simulink model "progetto_sim"  (R2025b)
settings: Solver=VariableStepAuto  StartTime=0.0  StopTime=1000  RelTol=1e-3
values from neighbouring files (symbols this model uses):
  d0 = [110 130 100 160]    [backup_id_macchine.mat]    (also in id_macchine.mat)
  dmin = 4    [backup_id_macchine.mat]    (also in id_macchine.mat)
  mDist = [156.727602966 155.419177889 157.307233343 156.111472907]    [backup_id_macchine.mat]    (also in id_macchine.mat = [156.911734511 155.758692096 157.721037406 156.538222818])
  t_cth = 3    [backup_id_macchine.mat]    (also in id_macchine.mat)
  Ts = 2    [backup_id_macchine.mat]    (also in id_macchine.mat)
  umax = 600    [backup_id_macchine.mat]    (also in id_macchine.mat)
  umin = -600    [backup_id_macchine.mat]    (also in id_macchine.mat)
  v0 = [10 12 15 9 10]    [backup_id_macchine.mat]    (also in id_macchine.mat)
  vMedio = [9.99088198605 9.9851530035 9.98261849858 9.98180014012]    [backup_id_macchine.mat]    (also in id_macchine.mat = [10.0026522625 10.0031571294 10.0027874656 10.0025052689])
  x0 = [10 12 15 9 10]    [backup_id_macchine.mat]    (also in id_macchine.mat)
undefined symbols (not defined in the file or in its folder): d1, d2, d3, d4, dspblkCoreblockFVToolHelper, gcbh, s2v2, s3v2, s4v2, s5v2
libraries: simulink x3, slctrl_signal x1
settings Model: Creator=david  LastModifiedBy=david

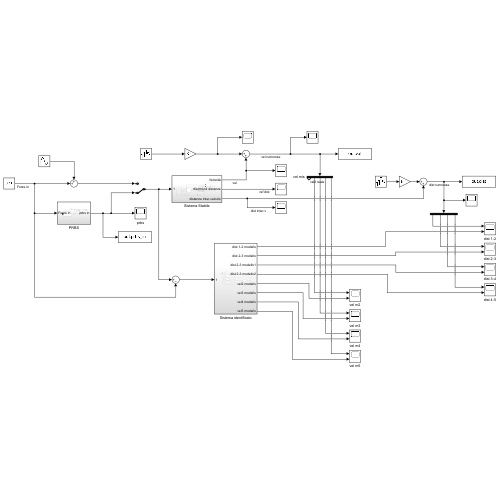
[thumbnail: Simulink's stored preview of the top-level diagram]
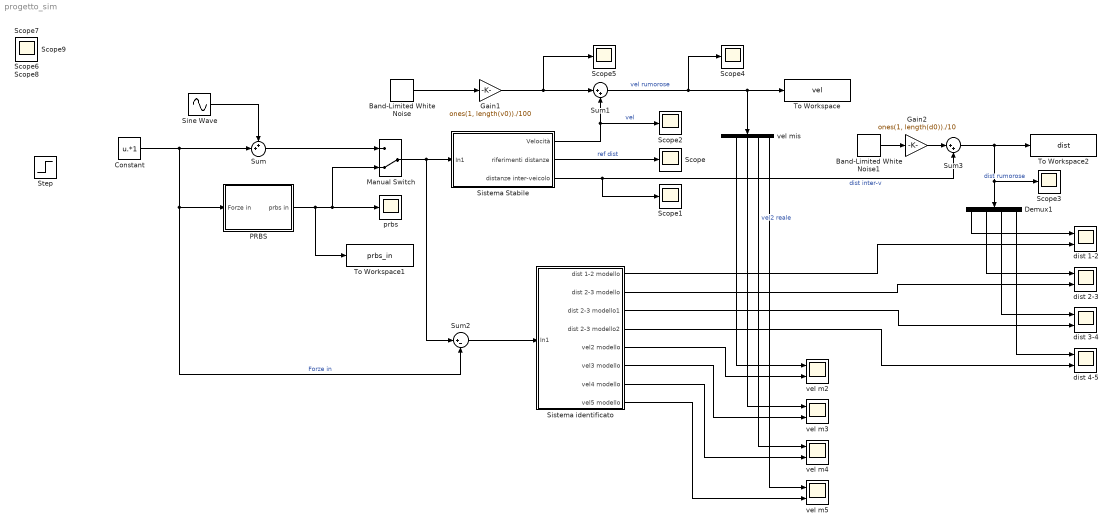
== system progetto_sim ==
  Band-Limited White Noise : simulink/Sources/Band-Limited White Noise  Cov=[0.1]  Ts=Ts  seed=[23341]
  Band-Limited White Noise1 : simulink/Sources/Band-Limited White Noise  Cov=[1]  Ts=Ts  seed=[23341]
  Constant : Constant  Value=u.*1
  Demux1 : Demux
  Gain1 : Gain  Gain=ones(1, length(v0))./100
  Gain2 : Gain  Gain=ones(1, length(d0))./10
  Manual Switch : ManualSwitch  CurrentSetting=0
  PRBS : Subsystem
  Scope{,1..9} (10 alike) : Scope
      Scope settings: ActiveDisplayYMinimum=20.100363251641021  ActiveDisplayYMaximum=52.211070749817665
      Scope1 settings: ActiveDisplayYMinimum=35.235374296085496  ActiveDisplayYMaximum=173.86273618932384
      Scope2 settings: ActiveDisplayYMinimum=6.4422971340740105  ActiveDisplayYMaximum=15.950855873991777  DataLoggingVariableName=ScopeData2
      Scope3 settings: ActiveDisplayYMinimum=92.525209670658455  ActiveDisplayYMaximum=167.52520967065848  DataLoggingVariableName=ScopeData14
      Scope4 settings: ActiveDisplayYMinimum=9.8362288071798236  ActiveDisplayYMaximum=10.170578899314256  DataLoggingVariableName=ScopeData4
      Scope5 settings: ActiveDisplayYMinimum=-0.1267870720741664  ActiveDisplayYMaximum=0.036491587322560859  DataLoggingVariableName=ScopeData5
      Scope6 settings: ActiveDisplayYMinimum=8.25  ActiveDisplayYMaximum=15.75  DataLoggingVariableName=ScopeData6
      Scope7 settings: ActiveDisplayYMinimum=5.9228633166114335  ActiveDisplayYMaximum=16.008570742598728  DataLoggingVariableName=ScopeData7
      Scope8 settings: ActiveDisplayYMinimum=-2.992302808171373  ActiveDisplayYMaximum=54.776922534241265  DataLoggingVariableName=ScopeData8
      Scope9 settings: ActiveDisplayYMinimum=90.6379126307081  ActiveDisplayYMaximum=184.25878632362713  DataLoggingVariableName=ScopeData9
  Sine Wave : Sin  Amplitude=10  Frequency=0.2  SampleTime=0
  Sistema Stabile : Subsystem
  Sistema identificato : Subsystem
  Sum : Sum  Inputs=++|
  Sum1 : Sum  Inputs=|++
  Sum2 : Sum  Inputs=|+-
  Sum3 : Sum  Inputs=|++
  To Workspace : ToWorkspace  VariableName=vel  SaveFormat=Timeseries  SampleTime=-1
  To Workspace1 : ToWorkspace  VariableName=prbs_in  SaveFormat=Timeseries  SampleTime=-1
  To Workspace2 : ToWorkspace  VariableName=dist  SaveFormat=Timeseries  SampleTime=-1
  dist 1-2 : Scope  NumInputPorts=2
      settings: ActiveDisplayYMinimum=97.650868190944664  ActiveDisplayYMaximum=163.45073412485041  DataLoggingVariableName=ScopeData15
  dist 2-3 : Scope  NumInputPorts=2
      settings: ActiveDisplayYMinimum=151.37082146304331  ActiveDisplayYMaximum=158.01387737377863  DataLoggingVariableName=ScopeData16
  dist 3-4 : Scope  NumInputPorts=2
      settings: ActiveDisplayYMinimum=92.836595832064589  ActiveDisplayYMaximum=164.47063751141872  DataLoggingVariableName=ScopeData17
  dist 4-5 : Scope  NumInputPorts=2
      settings: ActiveDisplayYMinimum=110.87620427965803  ActiveDisplayYMaximum=165.45819952448244  DataLoggingVariableName=ScopeData19
  prbs : Scope
      settings: ActiveDisplayYMinimum=-15.929445985668631  ActiveDisplayYMaximum=126.42137316665607  DataLoggingVariableName=ScopeData3
  vel m{2..5} (4 alike) : Scope  NumInputPorts=2
      vel m2 settings: ActiveDisplayYMinimum=7.6126289452019691  ActiveDisplayYMaximum=12.488371450292487  DataLoggingVariableName=ScopeData10
      vel m3 settings: ActiveDisplayYMinimum=5.38597542076137  ActiveDisplayYMaximum=16.068505060700495  DataLoggingVariableName=ScopeData11
      vel m4 settings: ActiveDisplayYMinimum=6.3078982373967136  ActiveDisplayYMaximum=10.954126895563874  DataLoggingVariableName=ScopeData12
      vel m5 settings: ActiveDisplayYMinimum=7.0228187670335016  ActiveDisplayYMaximum=11.300970971496861  DataLoggingVariableName=ScopeData13
  vel mis : Demux  Outputs=5
  Step : Step  IOType=siggen  SampleTime=0
  wires:
  Sistema Stabile/1(Velocità) -> Scope2/1, Sum1/2  "vel"
  Sistema Stabile/2(riferimenti distanze) -> Scope/1  "ref dist"
  Sistema Stabile/3(distanze inter-veicolo) -> Scope1/1, Sum3/2  "dist inter-v"
  Sum1/1 -> vel mis/1, To Workspace/1, Scope4/1  "vel rumorose"
  Constant/1 -> Sum2/2, PRBS/1(Forze in), Sum/2  "Forze in"
  Gain1/1 -> Sum1/1, Scope5/1
  PRBS/1(prbs in) -> Manual Switch/2, prbs/1, To Workspace1/1
  vel mis/3 -> vel m3/1
  vel mis/4 -> vel m4/1  "vel2 reale"
  vel mis/5 -> vel m5/1
  Band-Limited White Noise/1 -> Gain1/1
  Band-Limited White Noise1/1 -> Gain2/1
  Gain2/1 -> Sum3/1
  Sum3/1 -> To Workspace2/1, Scope3/1, Demux1/1  "dist rumorose"
  Demux1/1 -> dist 1-2/1
  vel mis/2 -> vel m2/1
  Sum/1 -> Manual Switch/1
  Demux1/2 -> dist 2-3/1
  Demux1/3 -> dist 3-4/1
  Demux1/4 -> dist 4-5/1
  Manual Switch/1 -> Sum2/1, Sistema Stabile/1(In1)
  Sistema identificato/1(dist 1-2 modello) -> dist 1-2/2
  Sistema identificato/2(dist 2-3 modello) -> dist 2-3/2
  Sistema identificato/5(vel2 modello) -> vel m2/2
  Sistema identificato/3(dist 2-3 modello1) -> dist 3-4/2
  Sistema identificato/4(dist 2-3 modello2) -> dist 4-5/2
  Sistema identificato/6(vel3 modello) -> vel m3/2
  Sistema identificato/7(vel4 modello) -> vel m4/2
  Sistema identificato/8(vel5 modello) -> vel m5/2
  Sum2/1 -> Sistema identificato/1(In1)
  Sine Wave/1 -> Sum/1

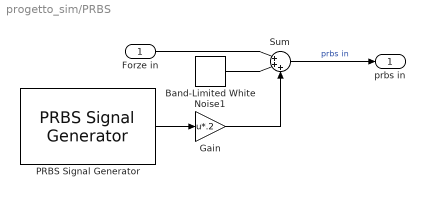
== system progetto_sim/PRBS ==
  Forze in : Inport
  Band-Limited White Noise1 : simulink/Sources/Band-Limited White Noise  Cov=[1]  Ts=Ts  seed=[23341]
  Gain : Gain  Gain=u*.2
  PRBS Signal Generator : slctrl_signal/PRBS Signal Generator  DiscreteTs=Ts  BlockDataType=double  SignalSource=Block parameters  Frequencies=[0.002 .007 .02]  FreqUnits=Hz  Amplitudes=1  NumOfFreq=3  NumOfPRBSPeriod=1  UseAutogenNumOfPRBSPeriod=off  PRBSSignalOrder=9  UseAutogenPRBSSignalOrder=off  UseExternalTs=off  CompiledTsChoice=InternalTs
      settings: LibrarySourceBlock=slctrlblks/Signal Generation/PRBS Signal Generator
  Sum : Sum  Inputs=|+++
  prbs in : Outport
  wires:
  Band-Limited White Noise1/1 -> Sum/2
  Sum/1 -> prbs in/1  "prbs in"
  PRBS Signal Generator/1 -> Gain/1
  Gain/1 -> Sum/3
  Forze in/1 -> Sum/1

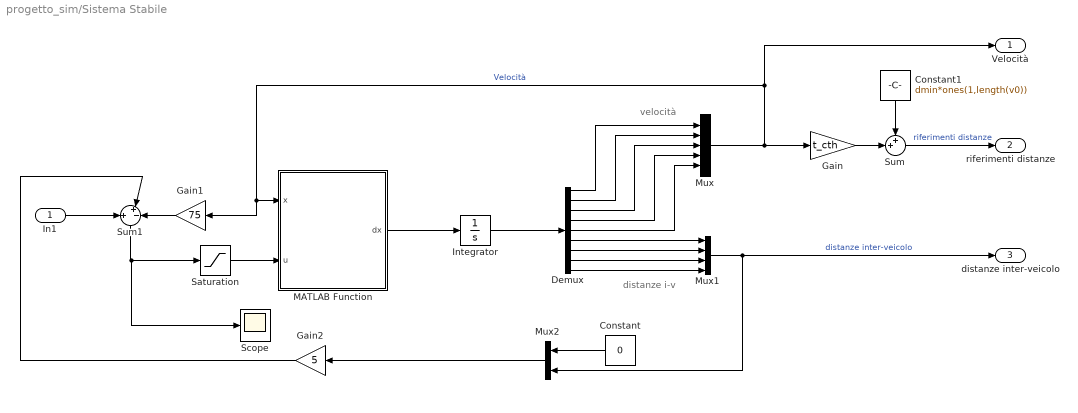
== system progetto_sim/Sistema Stabile ==
  note: distanze i-v
  note: velocità
  In1 : Inport
  Constant : Constant  Value=0
  Constant1 : Constant  Value=dmin*ones(1,length(v0))
  Demux : Demux  Outputs=9
  Gain : Gain  Gain=t_cth
  Gain1 : Gain  Gain=75
  Gain2 : Gain  Gain=5
  Integrator : Integrator  InitialCondition=[x0,d0]
  MATLAB Function : MATLAB Function  TreatAsAtomicUnit=on
  Mux : Mux  Inputs=5
  Mux1 : Mux
  Mux2 : Mux  Inputs=2
  Saturation : Saturate  UpperLimit=umax  LowerLimit=umin
  Scope : Scope
      settings: ActiveDisplayYMinimum=-870.07079552701  ActiveDisplayYMaximum=313.69351903872894  DataLoggingVariableName=ScopeData18
  Sum : Sum  Inputs=++|
  Sum1 : Sum  Inputs=+|+-
  Velocità : Outport
  riferimenti distanze : Outport  Port=2
  distanze inter-veicolo : Outport  Port=3
  wires:
  Mux/1 -> Gain1/1, MATLAB Function/1(x), Velocità/1, Gain/1  "Velocità"
  Demux/6 -> Mux1/1
  Saturation/1 -> MATLAB Function/2(u)
  Demux/4 -> Mux/4
  Integrator/1 -> Demux/1
  Demux/1 -> Mux/1
  Demux/8 -> Mux1/3
  Demux/3 -> Mux/3
  MATLAB Function/1(dx) -> Integrator/1
  Demux/2 -> Mux/2
  Demux/7 -> Mux1/2
  Demux/5 -> Mux/5
  Gain/1 -> Sum/2
  Constant1/1 -> Sum/1
  Sum1/1 -> Scope/1, Saturation/1
  Demux/9 -> Mux1/4
  Sum/1 -> riferimenti distanze/1  "riferimenti distanze"
  Mux1/1 -> Mux2/2, distanze inter-veicolo/1  "distanze inter-veicolo"
  In1/1 -> Sum1/1
  Constant/1 -> Mux2/1
  Mux2/1 -> Gain2/1
  Gain1/1 -> Sum1/3
  Gain2/1 -> Sum1/2

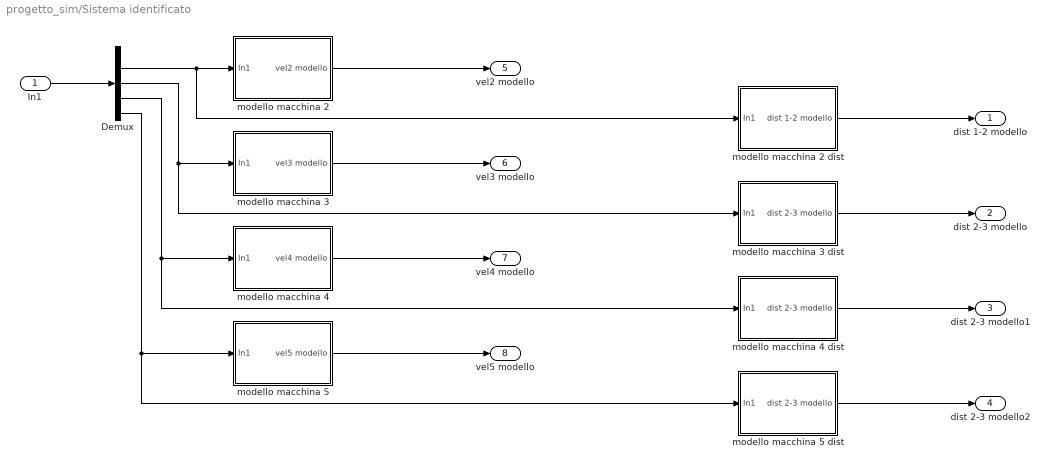
== system progetto_sim/Sistema identificato ==
  In1 : Inport
  Demux : Demux  Outputs=5
  modello macchina 2 : Subsystem
  modello macchina 2 dist : Subsystem
  modello macchina 3 : Subsystem
  modello macchina 3 dist : Subsystem
  modello macchina 4 : Subsystem
  modello macchina 4 dist : Subsystem
  modello macchina 5 : Subsystem
  modello macchina 5 dist : Subsystem
  dist 1-2 modello : Outport
  dist 2-3 modello : Outport  Port=2
  dist 2-3 modello1 : Outport  Port=3
  dist 2-3 modello2 : Outport  Port=4
  vel2 modello : Outport  Port=5
  vel3 modello : Outport  Port=6
  vel4 modello : Outport  Port=7
  vel5 modello : Outport  Port=8
  wires:
  modello macchina 2 dist/1(dist 1-2 modello) -> dist 1-2 modello/1
  modello macchina 2/1(vel2 modello) -> vel2 modello/1
  Demux/4 -> modello macchina 4/1(In1), modello macchina 4 dist/1(In1)
  modello macchina 4 dist/1(dist 2-3 modello) -> dist 2-3 modello1/1
  modello macchina 3 dist/1(dist 2-3 modello) -> dist 2-3 modello/1
  modello macchina 4/1(vel4 modello) -> vel4 modello/1
  Demux/5 -> modello macchina 5/1(In1), modello macchina 5 dist/1(In1)
  modello macchina 3/1(vel3 modello) -> vel3 modello/1
  Demux/2 -> modello macchina 2 dist/1(In1), modello macchina 2/1(In1)
  Demux/3 -> modello macchina 3/1(In1), modello macchina 3 dist/1(In1)
  modello macchina 5 dist/1(dist 2-3 modello) -> dist 2-3 modello2/1
  modello macchina 5/1(vel5 modello) -> vel5 modello/1
  In1/1 -> Demux/1

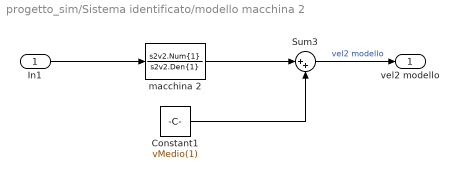
== system progetto_sim/Sistema identificato/modello macchina 2 ==
  In1 : Inport
  Constant1 : Constant  Value=vMedio(1)
  Sum3 : Sum  Inputs=|++
  macchina 2 : DiscreteFilter  LoadFcn=dspblkCoreblockFVToolHelper(gcbh,'load');  Numerator=s2v2.Num{1}  Denominator=s2v2.Den{1}
      settings: CopyFcn=dspblkCoreblockFVToolHelper(gcbh,'copy');  DeleteFcn=dspblkCoreblockFVToolHelper(gcbh,'close');  ModelCloseFcn=dspblkCoreblockFVToolHelper(gcbh,'close');  PreSaveFcn=dspblkCoreblockFVToolHelper(gcbh,'presave');  PostSaveFcn=dspblkCoreblockFVToolHelper(gcbh,'postsave');  CloseFcn=dspblkCoreblockFVToolHelper(gcbh,'close');
  vel2 modello : Outport
  wires:
  macchina 2/1 -> Sum3/1
  In1/1 -> macchina 2/1
  Constant1/1 -> Sum3/2
  Sum3/1 -> vel2 modello/1  "vel2 modello"

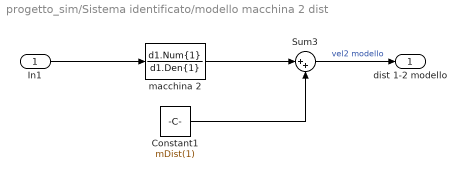
== system progetto_sim/Sistema identificato/modello macchina 2 dist ==
  In1 : Inport
  Constant1 : Constant  Value=mDist(1)
  Sum3 : Sum  Inputs=|++
  macchina 2 : DiscreteFilter  LoadFcn=dspblkCoreblockFVToolHelper(gcbh,'load');  Numerator=d1.Num{1}  Denominator=d1.Den{1}
      settings: CopyFcn=dspblkCoreblockFVToolHelper(gcbh,'copy');  DeleteFcn=dspblkCoreblockFVToolHelper(gcbh,'close');  ModelCloseFcn=dspblkCoreblockFVToolHelper(gcbh,'close');  PreSaveFcn=dspblkCoreblockFVToolHelper(gcbh,'presave');  PostSaveFcn=dspblkCoreblockFVToolHelper(gcbh,'postsave');  CloseFcn=dspblkCoreblockFVToolHelper(gcbh,'close');
  dist 1-2 modello : Outport
  wires:
  Sum3/1 -> dist 1-2 modello/1  "vel2 modello"
  Constant1/1 -> Sum3/2
  In1/1 -> macchina 2/1
  macchina 2/1 -> Sum3/1

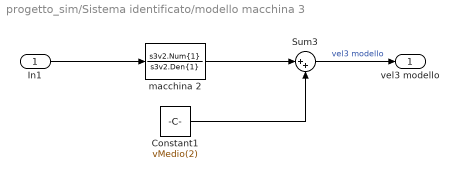
== system progetto_sim/Sistema identificato/modello macchina 3 ==
  In1 : Inport
  Constant1 : Constant  Value=vMedio(2)
  Sum3 : Sum  Inputs=|++
  macchina 2 : DiscreteFilter  LoadFcn=dspblkCoreblockFVToolHelper(gcbh,'load');  Numerator=s3v2.Num{1}  Denominator=s3v2.Den{1}
      settings: CopyFcn=dspblkCoreblockFVToolHelper(gcbh,'copy');  DeleteFcn=dspblkCoreblockFVToolHelper(gcbh,'close');  ModelCloseFcn=dspblkCoreblockFVToolHelper(gcbh,'close');  PreSaveFcn=dspblkCoreblockFVToolHelper(gcbh,'presave');  PostSaveFcn=dspblkCoreblockFVToolHelper(gcbh,'postsave');  CloseFcn=dspblkCoreblockFVToolHelper(gcbh,'close');
  vel3 modello : Outport
  wires:
  Sum3/1 -> vel3 modello/1  "vel3 modello"
  Constant1/1 -> Sum3/2
  In1/1 -> macchina 2/1
  macchina 2/1 -> Sum3/1

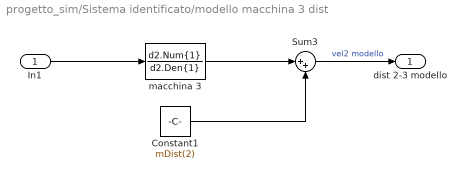
== system progetto_sim/Sistema identificato/modello macchina 3 dist ==
  In1 : Inport
  Constant1 : Constant  Value=mDist(2)
  Sum3 : Sum  Inputs=|++
  macchina 3 : DiscreteFilter  LoadFcn=dspblkCoreblockFVToolHelper(gcbh,'load');  Numerator=d2.Num{1}  Denominator=d2.Den{1}
      settings: CopyFcn=dspblkCoreblockFVToolHelper(gcbh,'copy');  DeleteFcn=dspblkCoreblockFVToolHelper(gcbh,'close');  ModelCloseFcn=dspblkCoreblockFVToolHelper(gcbh,'close');  PreSaveFcn=dspblkCoreblockFVToolHelper(gcbh,'presave');  PostSaveFcn=dspblkCoreblockFVToolHelper(gcbh,'postsave');  CloseFcn=dspblkCoreblockFVToolHelper(gcbh,'close');
  dist 2-3 modello : Outport
  wires:
  macchina 3/1 -> Sum3/1
  In1/1 -> macchina 3/1
  Constant1/1 -> Sum3/2
  Sum3/1 -> dist 2-3 modello/1  "vel2 modello"

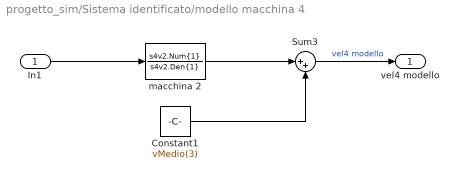
== system progetto_sim/Sistema identificato/modello macchina 4 ==
  In1 : Inport
  Constant1 : Constant  Value=vMedio(3)
  Sum3 : Sum  Inputs=|++
  macchina 2 : DiscreteFilter  LoadFcn=dspblkCoreblockFVToolHelper(gcbh,'load');  Numerator=s4v2.Num{1}  Denominator=s4v2.Den{1}
      settings: CopyFcn=dspblkCoreblockFVToolHelper(gcbh,'copy');  DeleteFcn=dspblkCoreblockFVToolHelper(gcbh,'close');  ModelCloseFcn=dspblkCoreblockFVToolHelper(gcbh,'close');  PreSaveFcn=dspblkCoreblockFVToolHelper(gcbh,'presave');  PostSaveFcn=dspblkCoreblockFVToolHelper(gcbh,'postsave');  CloseFcn=dspblkCoreblockFVToolHelper(gcbh,'close');
  vel4 modello : Outport
  wires:
  macchina 2/1 -> Sum3/1
  In1/1 -> macchina 2/1
  Constant1/1 -> Sum3/2
  Sum3/1 -> vel4 modello/1  "vel4 modello"

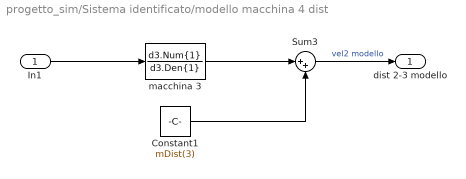
== system progetto_sim/Sistema identificato/modello macchina 4 dist ==
  In1 : Inport
  Constant1 : Constant  Value=mDist(3)
  Sum3 : Sum  Inputs=|++
  macchina 3 : DiscreteFilter  LoadFcn=dspblkCoreblockFVToolHelper(gcbh,'load');  Numerator=d3.Num{1}  Denominator=d3.Den{1}
      settings: CopyFcn=dspblkCoreblockFVToolHelper(gcbh,'copy');  DeleteFcn=dspblkCoreblockFVToolHelper(gcbh,'close');  ModelCloseFcn=dspblkCoreblockFVToolHelper(gcbh,'close');  PreSaveFcn=dspblkCoreblockFVToolHelper(gcbh,'presave');  PostSaveFcn=dspblkCoreblockFVToolHelper(gcbh,'postsave');  CloseFcn=dspblkCoreblockFVToolHelper(gcbh,'close');
  dist 2-3 modello : Outport
  wires:
  Sum3/1 -> dist 2-3 modello/1  "vel2 modello"
  Constant1/1 -> Sum3/2
  In1/1 -> macchina 3/1
  macchina 3/1 -> Sum3/1

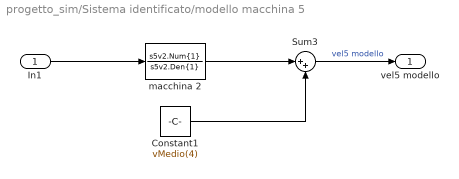
== system progetto_sim/Sistema identificato/modello macchina 5 ==
  In1 : Inport
  Constant1 : Constant  Value=vMedio(4)
  Sum3 : Sum  Inputs=|++
  macchina 2 : DiscreteFilter  LoadFcn=dspblkCoreblockFVToolHelper(gcbh,'load');  Numerator=s5v2.Num{1}  Denominator=s5v2.Den{1}
      settings: CopyFcn=dspblkCoreblockFVToolHelper(gcbh,'copy');  DeleteFcn=dspblkCoreblockFVToolHelper(gcbh,'close');  ModelCloseFcn=dspblkCoreblockFVToolHelper(gcbh,'close');  PreSaveFcn=dspblkCoreblockFVToolHelper(gcbh,'presave');  PostSaveFcn=dspblkCoreblockFVToolHelper(gcbh,'postsave');  CloseFcn=dspblkCoreblockFVToolHelper(gcbh,'close');
  vel5 modello : Outport
  wires:
  Sum3/1 -> vel5 modello/1  "vel5 modello"
  Constant1/1 -> Sum3/2
  In1/1 -> macchina 2/1
  macchina 2/1 -> Sum3/1

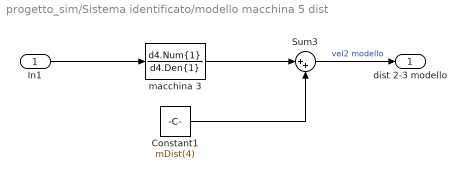
== system progetto_sim/Sistema identificato/modello macchina 5 dist ==
  In1 : Inport
  Constant1 : Constant  Value=mDist(4)
  Sum3 : Sum  Inputs=|++
  macchina 3 : DiscreteFilter  LoadFcn=dspblkCoreblockFVToolHelper(gcbh,'load');  Numerator=d4.Num{1}  Denominator=d4.Den{1}
      settings: CopyFcn=dspblkCoreblockFVToolHelper(gcbh,'copy');  DeleteFcn=dspblkCoreblockFVToolHelper(gcbh,'close');  ModelCloseFcn=dspblkCoreblockFVToolHelper(gcbh,'close');  PreSaveFcn=dspblkCoreblockFVToolHelper(gcbh,'presave');  PostSaveFcn=dspblkCoreblockFVToolHelper(gcbh,'postsave');  CloseFcn=dspblkCoreblockFVToolHelper(gcbh,'close');
  dist 2-3 modello : Outport
  wires:
  macchina 3/1 -> Sum3/1
  In1/1 -> macchina 3/1
  Constant1/1 -> Sum3/2
  Sum3/1 -> dist 2-3 modello/1  "vel2 modello"

== matlab function progetto_sim/Sistema Stabile/MATLAB Function ==
  data: x input; u input size=[1 5]; dx output size=[1 9]
function dx = sistemaVeicoli5(x, u)
% sistemaVeicoli5 - Modello dinamico 5 veicoli platooning
%
% Inputs:
%   t     - tempo (per integratori)
%   x     - stato: [v1, v2, v3, v4, v5, d2, d3, d4, d5]
%   u     - forze trazione [u1, u2, u3, u4, u5]
%
% Outputs:
%   dx    - derivata degli stati

m = [790 820 760 860 800];

rho = 1.22;        % Densità aria kg/m^3
caA = 0.88;        % Coeff Aerodinamico * superficie
cr = 0.01;         % Resistenza rotolamento stimata
gr = 9.81;         % Gravità

v = x(1:5);        % velocità
    
dv = zeros(1,5);
dd = zeros(1,4);

for i = 2:5
    FL = 0.5 * rho * caA * v(i)^2 + cr * m(i) * gr;
    dv(i) = (u(i) - FL) / m(i);

    dd(i-1) = v(i-1) - v(i);
end

dx = [dv'; dd']';

end
